simulink model "mass_spring_damper_system"  (R2018b)
settings: Solver=VariableStepAuto  StartTime=0.0  StopTime=30  RelTol=1e-3
InitFcn:
  | %%%%%%%%%%%%%%%%%%%%%%%%
  | %                  SYSTEM PARAMETERS             %
  | %%%%%%%%%%%%%%%%%%%%%%%%
  | 
  | m1 = 0.3;                       % Mass one value
  | m2 = 1;                     % Mass two value
  | k1 = 0.4;
  | k2 = 0.6;                          % Spring constant
  | fv1 = 0.7;
  | fv2 = 1;
  | b = 0.8;                          % Friction coefficient
settings Model: Creator=leony  LastModifiedBy=root
settings DebuggingCC: LibraryContextMissingDiagnostic=none
settings SFSimCC: SimUseLocalCustomCode=off
settings RTWCC: RTWUseLocalCustomCode=off

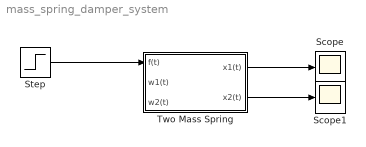
== system mass_spring_damper_system ==
  Scope : Scope
  Scope1 : Scope
  Step : Step  SampleTime=0
  Two Mass Spring : Subsystem
  wires:
  Two Mass Spring/1(x1(t)) -> Scope/1
  Two Mass Spring/2(x2(t)) -> Scope1/1
  Step/1 -> Two Mass Spring/1(f(t))

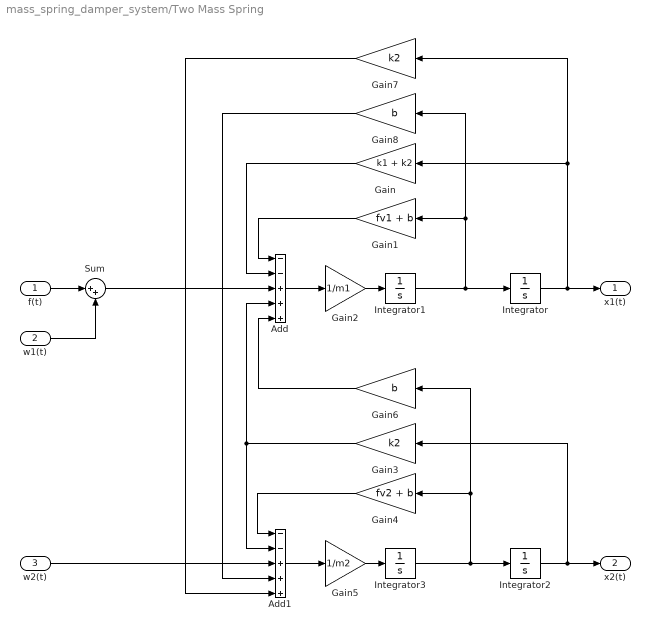
== system mass_spring_damper_system/Two Mass Spring ==
  f(t) : Inport
  w1(t) : Inport  Port=2
  w2(t) : Inport  Port=3
  Add : Sum  Inputs=--+++
  Add1 : Sum  Inputs=--+++
  Gain : Gain  Gain=k1 + k2
  Gain1 : Gain  Gain=fv1 + b
  Gain2 : Gain  Gain=1/m1
  Gain3 : Gain  Gain=k2
  Gain4 : Gain  Gain=fv2 + b
  Gain5 : Gain  Gain=1/m2
  Gain6 : Gain  Gain=b
  Gain7 : Gain  Gain=k2
  Gain8 : Gain  Gain=b
  Integrator : Integrator
  Integrator1 : Integrator
  Integrator2 : Integrator  InitialCondition=1
  Integrator3 : Integrator
  Sum : Sum  Inputs=|++
  x1(t) : Outport
  x2(t) : Outport  Port=2
  wires:
  w1(t)/1 -> Sum/2
  f(t)/1 -> Sum/1
  Integrator/1 -> Gain7/1, Gain/1, x1(t)/1
  Integrator1/1 -> Gain8/1, Gain1/1, Integrator/1
  Integrator3/1 -> Gain6/1, Gain4/1, Integrator2/1
  Integrator2/1 -> Gain3/1, x2(t)/1
  Gain2/1 -> Integrator1/1
  Add/1 -> Gain2/1
  Add1/1 -> Gain5/1
  Gain5/1 -> Integrator3/1
  Sum/1 -> Add/3
  Gain1/1 -> Add/1
  Gain/1 -> Add/2
  w2(t)/1 -> Add1/3
  Gain4/1 -> Add1/1
  Gain3/1 -> Add1/2, Add/4
  Gain6/1 -> Add/5
  Gain7/1 -> Add1/5
  Gain8/1 -> Add1/4
